simulink model "wiper_mdl_method2"  (R2024b)
settings: Solver=FixedStepDiscrete  StartTime=0.0  StopTime=20  FixedStep=10e-3  RelTol=1e-3
libraries: simulink x2, SignalEditorBlockLib x1
settings Model: Creator=Hassan Mohamed  LastModifiedBy=Hassan Mohamed

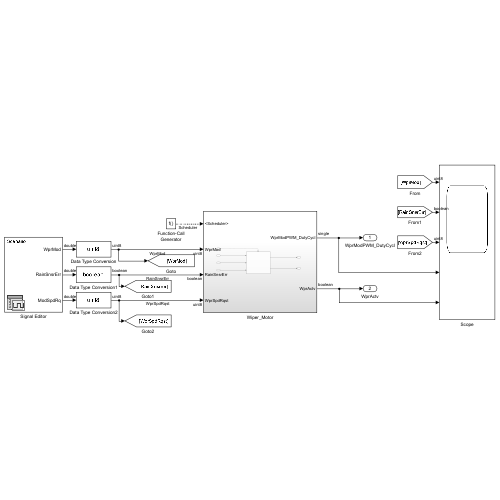
[thumbnail: Simulink's stored preview of the top-level diagram]
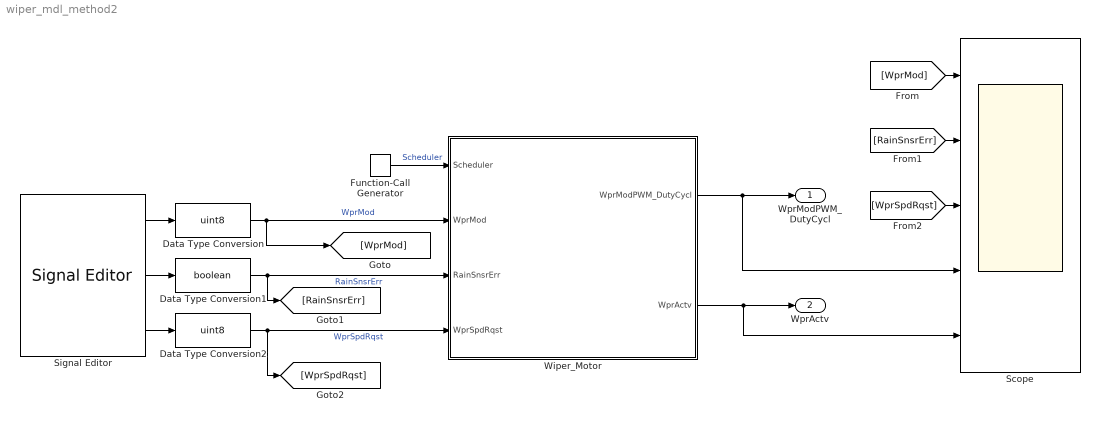
== system wiper_mdl_method2 ==
  Data Type Conversion : DataTypeConversion  OutMin=0  OutMax=3  OutDataTypeStr=uint8  SaturateOnIntegerOverflow=off  RndMeth=Floor
  Data Type Conversion1 : DataTypeConversion  OutDataTypeStr=boolean  SaturateOnIntegerOverflow=off  RndMeth=Floor
  Data Type Conversion2 : DataTypeConversion  OutDataTypeStr=uint8  SaturateOnIntegerOverflow=off  RndMeth=Floor
  Function-Call Generator : simulink/Ports & Subsystems/Function-Call Generator  sample_time=1  numberOfIterations=1  DisallowWideOutput=off
  Scope : Scope  NumInputPorts=5
  Signal Editor : SignalEditorBlockLib/Signal Editor  FileName=senario_2.mat  ActiveScenario=Scenario  ActiveSignal=WprMod  IsBus=off  OutputBusObjectStr=Bus: BusObject  SampleTime=0  Interpolate=off  ZeroCross=off  OutputAfterFinalValue=Setting to zero  Unit=inherit  PreserveSignalName=on  ApplySigPropsToAllScenarios=on  ApplySigPropsToAllSignals=on
  Wiper_Motor : Subsystem
  WprModPWM_DutyCycl : Outport
  WprActv : Outport  Port=2
  wires:
  Wiper_Motor/1(WprModPWM_DutyCycl) -> WprModPWM_DutyCycl/1, Scope/4
  Signal Editor/3 -> Data Type Conversion2/1
  Signal Editor/2 -> Data Type Conversion1/1
  Signal Editor/1 -> Data Type Conversion/1
  Wiper_Motor/2(WprActv) -> WprActv/1, Scope/5
  Function-Call Generator/1 -> Wiper_Motor/1(Scheduler)  "Scheduler"
  [RainSnsrErr] -> Scope/2
  [WprMod] -> Scope/1
  [WprSpdRqst] -> Scope/3
  Data Type Conversion/1 -> Wiper_Motor/2(WprMod), [WprMod]  "WprMod"
  Data Type Conversion1/1 -> Wiper_Motor/3(RainSnsrErr), [RainSnsrErr]  "RainSnsrErr"
  Data Type Conversion2/1 -> [WprSpdRqst], Wiper_Motor/4(WprSpdRqst)  "WprSpdRqst"

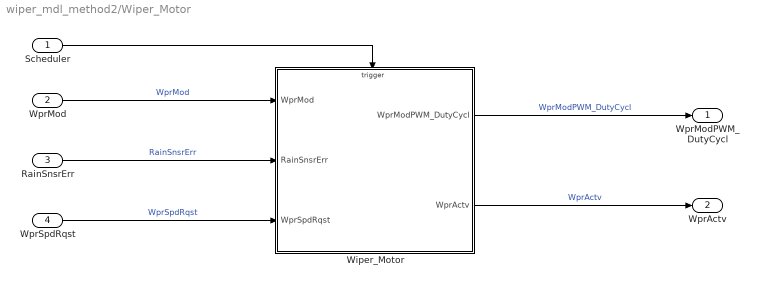
== system wiper_mdl_method2/Wiper_Motor ==
  Scheduler : Inport
  WprMod : Inport  Port=2  OutMin=0  OutMax=3  OutDataTypeStr=uint8
  RainSnsrErr : Inport  Port=3  OutMin=0  OutMax=1  OutDataTypeStr=boolean
  WprSpdRqst : Inport  Port=4  OutMin=0  OutMax=7  OutDataTypeStr=uint8
  Wiper_Motor : Subsystem  TreatAsAtomicUnit=on
  WprModPWM_DutyCycl : Outport
  WprActv : Outport  Port=2
  wires:
  Scheduler/1 -> Wiper_Motor/Trigger
  WprMod/1 -> Wiper_Motor/1(WprMod)  "WprMod"
  RainSnsrErr/1 -> Wiper_Motor/2(RainSnsrErr)  "RainSnsrErr"
  WprSpdRqst/1 -> Wiper_Motor/3(WprSpdRqst)  "WprSpdRqst"
  Wiper_Motor/1(WprModPWM_DutyCycl) -> WprModPWM_DutyCycl/1  "WprModPWM_DutyCycl"
  Wiper_Motor/2(WprActv) -> WprActv/1  "WprActv"

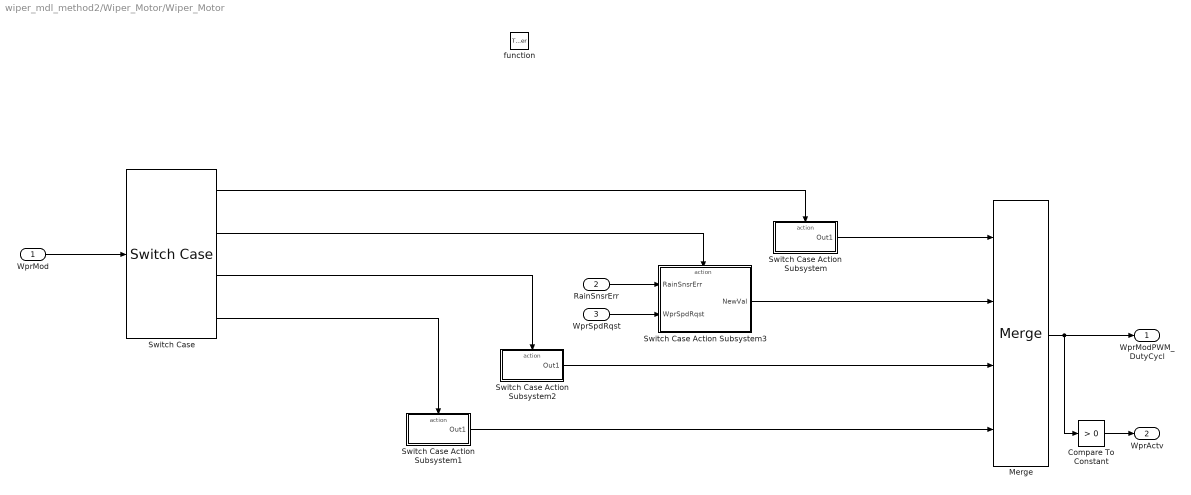
== system wiper_mdl_method2/Wiper_Motor/Wiper_Motor ==
  WprMod : Inport  OutMin=0  OutMax=3  OutDataTypeStr=uint8
  RainSnsrErr : Inport  Port=2  OutMin=0  OutMax=1  OutDataTypeStr=boolean
  WprSpdRqst : Inport  Port=3  OutMin=0  OutMax=7  OutDataTypeStr=uint8
  function : TriggerPort  TriggerType=function-call  VariantControl=(inherit)
  Compare To Constant : simulink/Logic and Bit Operations/Compare To Constant  relop=>  const=0  OutDataTypeStr=boolean
  Merge : Merge  Inputs=4
  Switch Case : SwitchCase  CaseConditions={0,1,2,3}  ShowDefaultCase=off
  Switch Case Action Subsystem : Subsystem  TreatAsAtomicUnit=on
  Switch Case Action Subsystem1 : Subsystem  TreatAsAtomicUnit=on
  Switch Case Action Subsystem2 : Subsystem  TreatAsAtomicUnit=on
  Switch Case Action Subsystem3 : Subsystem  TreatAsAtomicUnit=on
  WprModPWM_DutyCycl : Outport
  WprActv : Outport  Port=2
  wires:
  WprMod/1 -> Switch Case/1
  Switch Case/1 -> Switch Case Action Subsystem/Action
  Switch Case/4 -> Switch Case Action Subsystem1/Action
  Switch Case/3 -> Switch Case Action Subsystem2/Action
  Switch Case/2 -> Switch Case Action Subsystem3/Action
  WprSpdRqst/1 -> Switch Case Action Subsystem3/2(WprSpdRqst)
  RainSnsrErr/1 -> Switch Case Action Subsystem3/1(RainSnsrErr)
  Switch Case Action Subsystem/1(Out1) -> Merge/1
  Switch Case Action Subsystem2/1(Out1) -> Merge/3
  Switch Case Action Subsystem1/1(Out1) -> Merge/4
  Merge/1 -> WprModPWM_DutyCycl/1, Compare To Constant/1
  Compare To Constant/1 -> WprActv/1
  Switch Case Action Subsystem3/1(NewVal) -> Merge/2

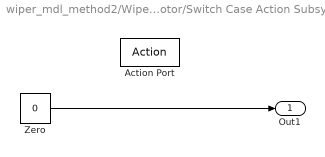
== system wiper_mdl_method2/Wiper_Motor/Wiper_Motor/Switch Case Action Subsystem ==
  Action Port : ActionPort  ActionPortLabel=case [ 0 ]:
  Zero : Constant  Value=0  OutDataTypeStr=Inherit: Inherit via back propagation
  Out1 : Outport
  wires:
  Zero/1 -> Out1/1

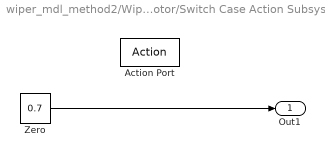
== system wiper_mdl_method2/Wiper_Motor/Wiper_Motor/Switch Case Action Subsystem1 ==
  Action Port : ActionPort  ActionPortLabel=case [ 3 ]:
  Zero : Constant  Value=0.7  OutDataTypeStr=Inherit: Inherit via back propagation
  Out1 : Outport
  wires:
  Zero/1 -> Out1/1

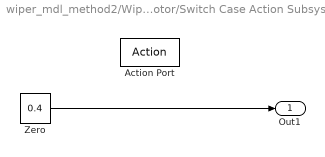
== system wiper_mdl_method2/Wiper_Motor/Wiper_Motor/Switch Case Action Subsystem2 ==
  Action Port : ActionPort  ActionPortLabel=case [ 2 ]:
  Zero : Constant  Value=0.4  OutDataTypeStr=Inherit: Inherit via back propagation
  Out1 : Outport
  wires:
  Zero/1 -> Out1/1

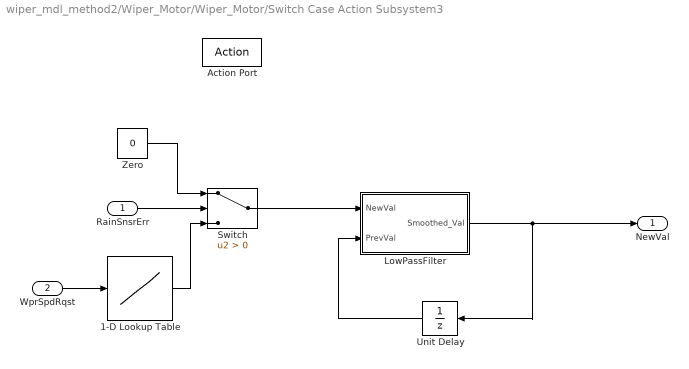
== system wiper_mdl_method2/Wiper_Motor/Wiper_Motor/Switch Case Action Subsystem3 ==
  RainSnsrErr : Inport
  WprSpdRqst : Inport  Port=2
  Action Port : ActionPort  ActionPortLabel=case [ 1 ]:
  1-D Lookup Table : Lookup_n-D  NumberOfTableDimensions=1  BreakpointsForDimension1=[0 1 2 3 4 5 6 7]  Table=[0 0.4 0.45 0.5 0.55 0.6 0.65 0.7]  TableDataTypeStr=single  ExtrapMethod=Clip  InternalRulePriority=Speed  OutDataTypeStr=single  RndMeth=Simplest
  LowPassFilter : Subsystem  TreatAsAtomicUnit=on
  Switch : Switch  Criteria=u2 > Threshold  SaturateOnIntegerOverflow=off  InputSameDT=off
  Unit Delay : UnitDelay  SampleTime=-1  HasFrameUpgradeWarning=on
  Zero : Constant  Value=0  OutDataTypeStr=Inherit: Inherit via back propagation
  NewVal : Outport
  wires:
  RainSnsrErr/1 -> Switch/2
  Zero/1 -> Switch/1
  Switch/1 -> LowPassFilter/1(NewVal)
  WprSpdRqst/1 -> 1-D Lookup Table/1
  1-D Lookup Table/1 -> Switch/3
  LowPassFilter/1(Smoothed_Val) -> NewVal/1, Unit Delay/1
  Unit Delay/1 -> LowPassFilter/2(PrevVal)

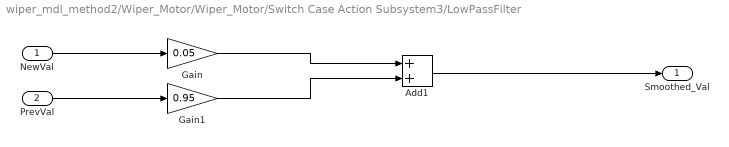
== system wiper_mdl_method2/Wiper_Motor/Wiper_Motor/Switch Case Action Subsystem3/LowPassFilter ==
  NewVal : Inport
  PrevVal : Inport  Port=2
  Add1 : Sum  OutDataTypeStr=single
  Gain : Gain  Gain=0.05
  Gain1 : Gain  Gain=0.95
  Smoothed_Val : Outport
  wires:
  PrevVal/1 -> Gain1/1
  NewVal/1 -> Gain/1
  Gain/1 -> Add1/1
  Gain1/1 -> Add1/2
  Add1/1 -> Smoothed_Val/1
